simulink model "Horloge_interne_v3"  (R2023a)
settings: Solver=VariableStepAuto  StartTime=0.0  StopTime=20  RelTol=1e-3
settings Model: Creator=Khalid-B  LastModifiedBy=Khalid-B

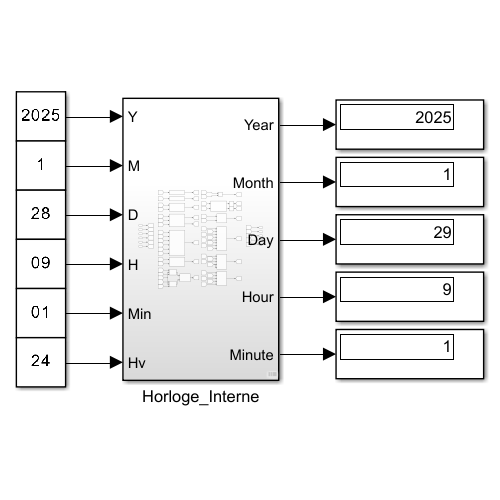
[thumbnail: Simulink's stored preview of the top-level diagram]
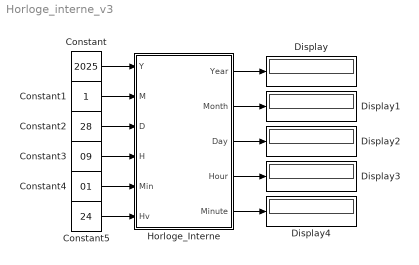
== system Horloge_interne_v3 ==
  Constant : Constant  Value=2025  OutDataTypeStr=uint32
  Constant1 : Constant  OutDataTypeStr=uint32
  Constant2 : Constant  Value=28  OutDataTypeStr=uint32
  Constant3 : Constant  Value=09  OutDataTypeStr=uint32
  Constant4 : Constant  Value=01  OutDataTypeStr=uint32
  Constant5 : Constant  Value=24  OutDataTypeStr=uint32
  Display{,1..4} (5 alike) : Display
  Horloge_Interne : Subsystem
  wires:
  Constant4/1 -> Horloge_Interne/5(Min)
  Constant2/1 -> Horloge_Interne/3(D)
  Horloge_Interne/4(Hour) -> Display3/1
  Horloge_Interne/2(Month) -> Display1/1
  Constant/1 -> Horloge_Interne/1(Y)
  Constant1/1 -> Horloge_Interne/2(M)
  Constant3/1 -> Horloge_Interne/4(H)
  Horloge_Interne/5(Minute) -> Display4/1
  Horloge_Interne/3(Day) -> Display2/1
  Horloge_Interne/1(Year) -> Display/1
  Constant5/1 -> Horloge_Interne/6(Hv)

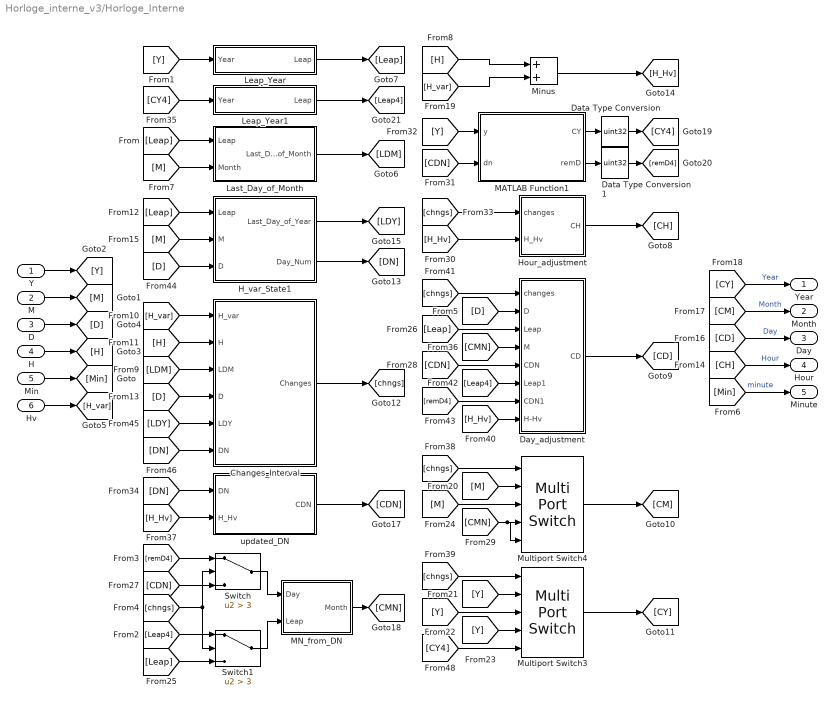
== system Horloge_interne_v3/Horloge_Interne ==
  Y : Inport
  M : Inport  Port=2
  D : Inport  Port=3
  H : Inport  Port=4
  Min : Inport  Port=5
  Hv : Inport  Port=6
  Changes_Interval : Subsystem
  Data Type Conversion : DataTypeConversion  OutDataTypeStr=uint32  SaturateOnIntegerOverflow=off  RndMeth=Floor
  Data Type Conversion1 : DataTypeConversion  OutDataTypeStr=uint32  SaturateOnIntegerOverflow=off  RndMeth=Floor
  Day_adjustment : Subsystem
  H_var_State1 : Subsystem
  Hour_adjustment : Subsystem
  Last_Day_of_Month : Subsystem
  Leap_Year : Subsystem
  Leap_Year1 : Subsystem
  MATLAB Function1 : MATLAB Function  TreatAsAtomicUnit=on
  MN_from_DN : Subsystem
  Minus : Sum
  Multiport Switch3 : MultiPortSwitch  Inputs=4  SaturateOnIntegerOverflow=off  InputSameDT=off
  Multiport Switch4 : MultiPortSwitch  Inputs=4  SaturateOnIntegerOverflow=off  InputSameDT=off
  Switch : Switch  Criteria=u2 > Threshold  Threshold=3  SaturateOnIntegerOverflow=off  InputSameDT=off
  Switch1 : Switch  Criteria=u2 > Threshold  Threshold=3  SaturateOnIntegerOverflow=off  InputSameDT=off
  updated_DN : Subsystem
  Year : Outport
  Month : Outport  Port=2
  Day : Outport  Port=3
  Hour : Outport  Port=4
  Minute : Outport  Port=5
  wires:
  updated_DN/1(CDN) -> [CDN]
  [CMN] -> Day_adjustment/4(M)
  [D] -> Day_adjustment/2(D)
  D/1 -> [D]
  [M] -> Last_Day_of_Month/2(Month)
  [H_Hv] -> Hour_adjustment/2(H_Hv)
  [H_Hv] -> updated_DN/2(H_Hv)
  [Y] -> Multiport Switch3/4
  [D] -> Changes_Interval/4(D)
  [Leap] -> H_var_State1/1(Leap)
  [CDN] -> Switch/3
  [H] -> Changes_Interval/2(H)
  M/1 -> [M]
  [Leap4] -> Switch1/1
  [chngs] -> Multiport Switch3/1
  [CDN] -> Day_adjustment/5(CDN)
  MATLAB Function1/1(CY) -> Data Type Conversion/1
  [Leap] -> Day_adjustment/3(Leap)
  [Y] -> Multiport Switch3/3
  MATLAB Function1/2(remD) -> Data Type Conversion1/1
  Changes_Interval/1(Changes) -> [chngs]
  Min/1 -> [Min]
  Multiport Switch4/1 -> [CM]
  [Leap4] -> Day_adjustment/6(Leap1)
  [H_var] -> Changes_Interval/1(H_var)
  Multiport Switch3/1 -> [CY]
  [remD4] -> Day_adjustment/7(CDN1)
  [CMN] -> Multiport Switch4/5, Multiport Switch4/4
  [chngs] -> Day_adjustment/1(changes)
  [chngs] -> Multiport Switch4/1
  [M] -> H_var_State1/2(M)
  [LDM] -> Changes_Interval/3(LDM)
  [Y] -> Multiport Switch3/2
  Last_Day_of_Month/1(Last_Day_of_Month) -> [LDM]
  [chngs] -> Switch/2, Switch1/2
  [M] -> Multiport Switch4/3
  [Leap] -> Switch1/3
  [DN] -> updated_DN/1(DN)
  [CDN] -> MATLAB Function1/2(dn)
  [M] -> Multiport Switch4/2
  MN_from_DN/1(Month) -> [CMN]
  [CY4] -> Multiport Switch3/5
  [Y] -> MATLAB Function1/1(y)
  Data Type Conversion1/1 -> [remD4]
  Day_adjustment/1(CD) -> [CD]
  [chngs] -> Hour_adjustment/1(changes)
  Hour_adjustment/1(CH) -> [CH]
  Data Type Conversion/1 -> [CY4]
  [remD4] -> Switch/1
  Y/1 -> [Y]
  [H_Hv] -> Day_adjustment/8(H-Hv)
  [Leap] -> Last_Day_of_Month/1(Leap)
  [CY] -> Year/1  "Year"
  [CM] -> Month/1  "Month"
  Hv/1 -> [H_var]
  [Min] -> Minute/1  "minute"
  H/1 -> [H]
  [CH] -> Hour/1  "Hour"
  [CD] -> Day/1  "Day"
  Leap_Year/1(Leap) -> [Leap]
  [Y] -> Leap_Year/1(Year)
  Leap_Year1/1(Leap) -> [Leap4]
  [CY4] -> Leap_Year1/1(Year)
  Switch/1 -> MN_from_DN/1(Day)
  Switch1/1 -> MN_from_DN/2(Leap)
  [D] -> H_var_State1/3(D)
  H_var_State1/2(Day_Num) -> [DN]
  H_var_State1/1(Last_Day_of_Year) -> [LDY]
  [LDY] -> Changes_Interval/5(LDY)
  [DN] -> Changes_Interval/6(DN)
  [H] -> Minus/1
  Minus/1 -> [H_Hv]
  [H_var] -> Minus/2

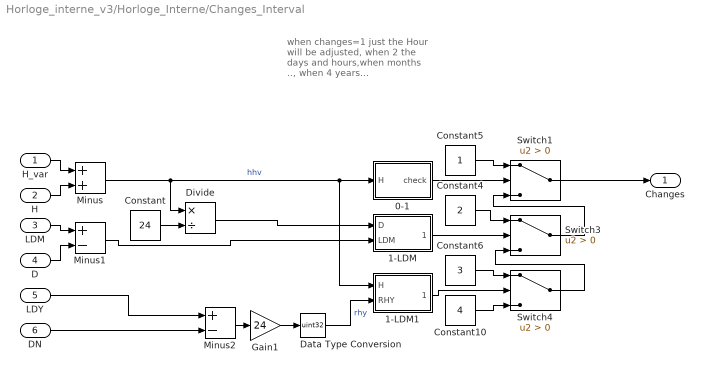
== system Horloge_interne_v3/Horloge_Interne/Changes_Interval ==
  note: when changes=1 just the Hour will be adjusted, when 2 the days and hours,when months .., when 4 years...
  H_var : Inport
  H : Inport  Port=2
  LDM : Inport  Port=3
  D : Inport  Port=4
  LDY : Inport  Port=5
  DN : Inport  Port=6
  0-1 : Subsystem
  1-LDM : Subsystem
  1-LDM1 : Subsystem
  Constant : Constant  Value=24  OutDataTypeStr=uint32
  Constant10 : Constant  Value=4  OutDataTypeStr=uint32
  Constant4 : Constant  Value=2  OutDataTypeStr=uint32
  Constant5 : Constant  OutDataTypeStr=uint32
  Constant6 : Constant  Value=3  OutDataTypeStr=uint32
  Data Type Conversion : DataTypeConversion  OutDataTypeStr=uint32  SaturateOnIntegerOverflow=off  RndMeth=Floor
  Divide : Product  Inputs=*/
  Gain1 : Gain  Gain=24
  Minus : Sum
  Minus1 : Sum  Inputs=+-
  Minus2 : Sum  Inputs=+-
  Switch1 : Switch  Criteria=u2 > Threshold  SaturateOnIntegerOverflow=off  InputSameDT=off
  Switch3 : Switch  Criteria=u2 > Threshold  SaturateOnIntegerOverflow=off  InputSameDT=off
  Switch4 : Switch  Criteria=u2 > Threshold  SaturateOnIntegerOverflow=off  InputSameDT=off
  Changes : Outport
  wires:
  Constant6/1 -> Switch4/1
  0-1/1(check) -> Switch1/2
  Constant5/1 -> Switch1/1
  Constant4/1 -> Switch3/1
  1-LDM/1(check) -> Switch3/2
  Minus/1 -> Divide/1, 0-1/1(H), 1-LDM1/1(H)  "hhv"
  Switch4/1 -> Switch3/3
  H/1 -> Minus/2
  1-LDM1/1(check) -> Switch4/2
  Constant10/1 -> Switch4/3
  Switch3/1 -> Switch1/3
  LDM/1 -> Minus1/1
  Minus2/1 -> Gain1/1
  H_var/1 -> Minus/1
  Switch1/1 -> Changes/1
  Constant/1 -> Divide/2
  Divide/1 -> 1-LDM/1(D)
  Data Type Conversion/1 -> 1-LDM1/2(RHY)  "rhy"
  Minus1/1 -> 1-LDM/2(LDM)
  Gain1/1 -> Data Type Conversion/1
  D/1 -> Minus1/2
  LDY/1 -> Minus2/1
  DN/1 -> Minus2/2

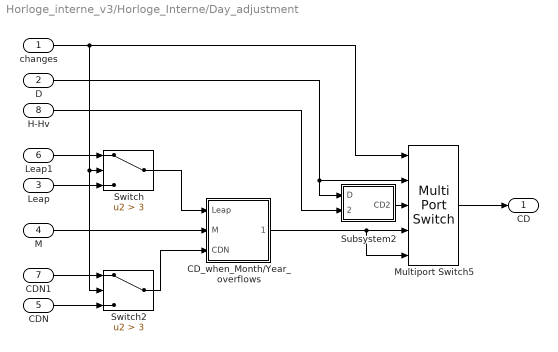
== system Horloge_interne_v3/Horloge_Interne/Day_adjustment ==
  changes : Inport
  D : Inport  Port=2
  Leap : Inport  Port=3
  M : Inport  Port=4
  CDN : Inport  Port=5
  Leap1 : Inport  Port=6
  CDN1 : Inport  Port=7
  H-Hv : Inport  Port=8
  CD_when_Month/Year_overflows : Subsystem
  Multiport Switch5 : MultiPortSwitch  Inputs=4  SaturateOnIntegerOverflow=off  InputSameDT=off
  Subsystem2 : Subsystem
  Switch : Switch  Criteria=u2 > Threshold  Threshold=3  SaturateOnIntegerOverflow=off  InputSameDT=off
  Switch2 : Switch  Criteria=u2 > Threshold  Threshold=3  SaturateOnIntegerOverflow=off  InputSameDT=off
  CD : Outport
  wires:
  changes/1 -> Switch2/2, Switch/2, Multiport Switch5/1
  Subsystem2/1(CD2) -> Multiport Switch5/3
  Multiport Switch5/1 -> CD/1
  D/1 -> Subsystem2/1(D), Multiport Switch5/2
  H-Hv/1 -> Subsystem2/2(H_Hv)
  CD_when_Month/Year_overflows/1(CD3_4) -> Multiport Switch5/5, Multiport Switch5/4
  Leap1/1 -> Switch/1
  Leap/1 -> Switch/3
  CDN1/1 -> Switch2/1
  CDN/1 -> Switch2/3
  M/1 -> CD_when_Month/Year_overflows/2(M)
  Switch/1 -> CD_when_Month/Year_overflows/1(Leap)
  Switch2/1 -> CD_when_Month/Year_overflows/3(CDN)

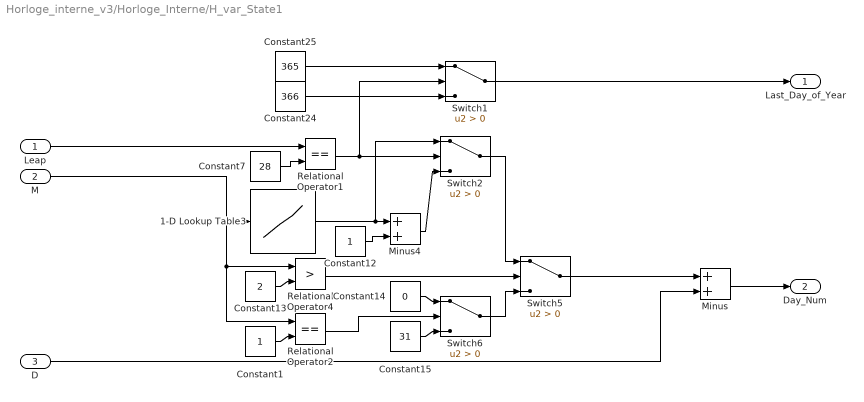
== system Horloge_interne_v3/Horloge_Interne/H_var_State1 ==
  Leap : Inport
  M : Inport  Port=2
  D : Inport  Port=3
  1-D Lookup Table3 : Lookup_n-D  NumberOfTableDimensions=1  BreakpointsSpecification=Even spacing  BreakpointsForDimension1=[-5:5]  Table=[0 0 59 90 120 151 181 212 243 273 304 334]  InterpMethod=Flat  InternalRulePriority=Speed  RndMeth=Simplest
  Constant1 : Constant  OutDataTypeStr=uint32
  Constant12 : Constant  OutDataTypeStr=uint32
  Constant13 : Constant  Value=2  OutDataTypeStr=uint32
  Constant14 : Constant  Value=0  OutDataTypeStr=uint32
  Constant15 : Constant  Value=31  OutDataTypeStr=uint32
  Constant24 : Constant  Value=366  OutDataTypeStr=uint32
  Constant25 : Constant  Value=365  OutDataTypeStr=uint32
  Constant7 : Constant  Value=28  OutDataTypeStr=uint32
  Minus : Sum
  Minus4 : Sum
  Relational Operator1 : RelationalOperator  Operator===  OutDataTypeStr=boolean  RndMeth=Simplest  InputSameDT=off
  Relational Operator2 : RelationalOperator  Operator===  OutDataTypeStr=boolean  RndMeth=Simplest  InputSameDT=off
  Relational Operator4 : RelationalOperator  Operator=>  OutDataTypeStr=boolean  RndMeth=Simplest  InputSameDT=off
  Switch{1..2,5..6} (4 alike) : Switch  Criteria=u2 > Threshold  SaturateOnIntegerOverflow=off  InputSameDT=off
  Last_Day_of_Year : Outport
  Day_Num : Outport  Port=2
  wires:
  M/1 -> Relational Operator2/1, Relational Operator4/1, 1-D Lookup Table3/1
  Switch1/1 -> Last_Day_of_Year/1
  Constant24/1 -> Switch1/3
  Constant25/1 -> Switch1/1
  Switch5/1 -> Minus/1
  D/1 -> Minus/2
  Minus/1 -> Day_Num/1
  Constant15/1 -> Switch6/3
  Constant12/1 -> Minus4/2
  Relational Operator4/1 -> Switch5/2
  Minus4/1 -> Switch2/3
  Switch2/1 -> Switch5/1
  Relational Operator1/1 -> Switch2/2, Switch1/2
  Constant13/1 -> Relational Operator4/2
  1-D Lookup Table3/1 -> Switch2/1, Minus4/1
  Constant7/1 -> Relational Operator1/2
  Switch6/1 -> Switch5/3
  Constant14/1 -> Switch6/1
  Leap/1 -> Relational Operator1/1
  Constant1/1 -> Relational Operator2/2
  Relational Operator2/1 -> Switch6/2

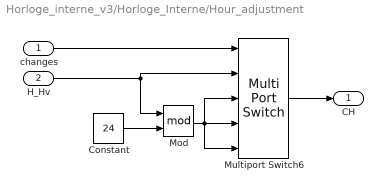
== system Horloge_interne_v3/Horloge_Interne/Hour_adjustment ==
  changes : Inport
  H_Hv : Inport  Port=2
  Constant : Constant  Value=24  OutDataTypeStr=uint32
  Mod : Math  Operator=mod
  Multiport Switch6 : MultiPortSwitch  Inputs=4  SaturateOnIntegerOverflow=off  InputSameDT=off
  CH : Outport
  wires:
  Multiport Switch6/1 -> CH/1
  H_Hv/1 -> Mod/1, Multiport Switch6/2
  Constant/1 -> Mod/2
  Mod/1 -> Multiport Switch6/5, Multiport Switch6/3, Multiport Switch6/4
  changes/1 -> Multiport Switch6/1

== system Horloge_interne_v3/Horloge_Interne/Last_Day_of_Month ==
  Leap : Inport
  Month : Inport  Port=2
  1-D Lookup Table : Lookup_n-D  NumberOfTableDimensions=1  LookupTableObject=obj1  BreakpointsSpecification=Even spacing  BreakpointsForDimension1=[1 3 5 6]  Table=[31 28 31 30 31 30 31 31 30 31 30 31]  InterpMethod=Flat  InternalRulePriority=Speed  RndMeth=Simplest
  Switch : Switch  Criteria=u2 > Threshold  Threshold=28  SaturateOnIntegerOverflow=off  InputSameDT=off
  Last_Day_of_Month : Outport
  wires:
  Leap/1 -> Switch/1, Switch/2
  Month/1 -> 1-D Lookup Table/1
  Switch/1 -> Last_Day_of_Month/1  "Last_Day_of_Month"
  1-D Lookup Table/1 -> Switch/3

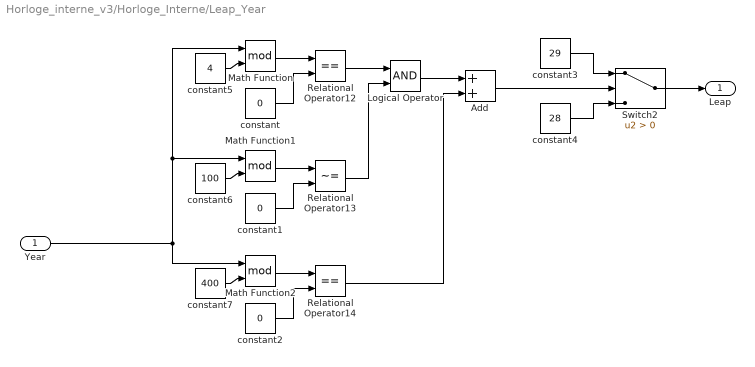
== system Horloge_interne_v3/Horloge_Interne/Leap_Year ==
  Year : Inport
  Add : Sum
  Logical Operator : Logic  AllPortsSameDT=off  OutDataTypeStr=boolean
  Math Function : Math  Operator=mod
  Math Function1 : Math  Operator=mod
  Math Function2 : Math  Operator=mod
  Relational Operator12 : RelationalOperator  Operator===  OutDataTypeStr=boolean  RndMeth=Simplest  InputSameDT=off
  Relational Operator13 : RelationalOperator  Operator=~=  OutDataTypeStr=boolean  RndMeth=Simplest  InputSameDT=off
  Relational Operator14 : RelationalOperator  Operator===  OutDataTypeStr=boolean  RndMeth=Simplest  InputSameDT=off
  Switch2 : Switch  Criteria=u2 > Threshold  SaturateOnIntegerOverflow=off  InputSameDT=off
  constant : Constant  Value=0  OutDataTypeStr=uint32
  constant1 : Constant  Value=0  OutDataTypeStr=uint32
  constant2 : Constant  Value=0  OutDataTypeStr=uint32
  constant3 : Constant  Value=29  OutDataTypeStr=uint32
  constant4 : Constant  Value=28  OutDataTypeStr=uint32
  constant5 : Constant  Value=4  OutDataTypeStr=uint32
  constant6 : Constant  Value=100  OutDataTypeStr=uint32
  constant7 : Constant  Value=400  OutDataTypeStr=uint32
  Leap : Outport
  wires:
  constant/1 -> Relational Operator12/2
  constant4/1 -> Switch2/3
  Year/1 -> Math Function2/1, Math Function1/1, Math Function/1
  Switch2/1 -> Leap/1
  Math Function2/1 -> Relational Operator14/1
  Relational Operator12/1 -> Logical Operator/1
  constant5/1 -> Math Function/2
  Relational Operator14/1 -> Add/2
  constant2/1 -> Relational Operator14/2
  Math Function/1 -> Relational Operator12/1
  Logical Operator/1 -> Add/1
  constant1/1 -> Relational Operator13/2
  Add/1 -> Switch2/2
  Relational Operator13/1 -> Logical Operator/2
  constant3/1 -> Switch2/1
  constant6/1 -> Math Function1/2
  constant7/1 -> Math Function2/2
  Math Function1/1 -> Relational Operator13/1

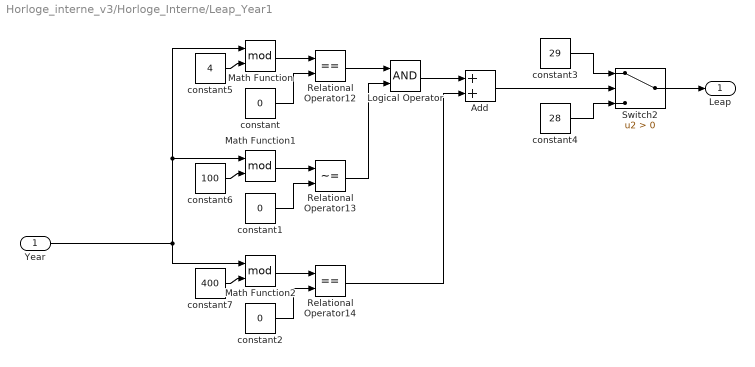
== system Horloge_interne_v3/Horloge_Interne/Leap_Year1 ==
  Year : Inport
  Add : Sum
  Logical Operator : Logic  AllPortsSameDT=off  OutDataTypeStr=boolean
  Math Function : Math  Operator=mod
  Math Function1 : Math  Operator=mod
  Math Function2 : Math  Operator=mod
  Relational Operator12 : RelationalOperator  Operator===  OutDataTypeStr=boolean  RndMeth=Simplest  InputSameDT=off
  Relational Operator13 : RelationalOperator  Operator=~=  OutDataTypeStr=boolean  RndMeth=Simplest  InputSameDT=off
  Relational Operator14 : RelationalOperator  Operator===  OutDataTypeStr=boolean  RndMeth=Simplest  InputSameDT=off
  Switch2 : Switch  Criteria=u2 > Threshold  SaturateOnIntegerOverflow=off  InputSameDT=off
  constant : Constant  Value=0  OutDataTypeStr=uint32
  constant1 : Constant  Value=0  OutDataTypeStr=uint32
  constant2 : Constant  Value=0  OutDataTypeStr=uint32
  constant3 : Constant  Value=29  OutDataTypeStr=uint32
  constant4 : Constant  Value=28  OutDataTypeStr=uint32
  constant5 : Constant  Value=4  OutDataTypeStr=uint32
  constant6 : Constant  Value=100  OutDataTypeStr=uint32
  constant7 : Constant  Value=400  OutDataTypeStr=uint32
  Leap : Outport
  wires:
  constant/1 -> Relational Operator12/2
  constant4/1 -> Switch2/3
  Year/1 -> Math Function2/1, Math Function1/1, Math Function/1
  Switch2/1 -> Leap/1
  Math Function2/1 -> Relational Operator14/1
  Relational Operator12/1 -> Logical Operator/1
  constant5/1 -> Math Function/2
  Relational Operator14/1 -> Add/2
  constant2/1 -> Relational Operator14/2
  Math Function/1 -> Relational Operator12/1
  Logical Operator/1 -> Add/1
  constant1/1 -> Relational Operator13/2
  Add/1 -> Switch2/2
  Relational Operator13/1 -> Logical Operator/2
  constant3/1 -> Switch2/1
  constant6/1 -> Math Function1/2
  constant7/1 -> Math Function2/2
  Math Function1/1 -> Relational Operator13/1

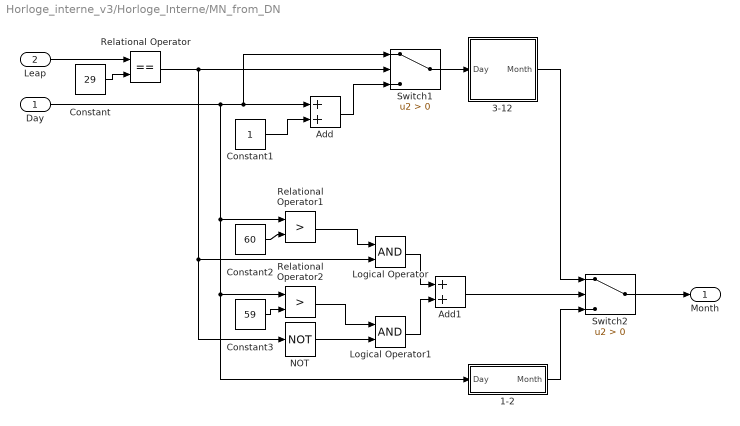
== system Horloge_interne_v3/Horloge_Interne/MN_from_DN ==
  Day : Inport
  Leap : Inport  Port=2
  1-2 : Subsystem
  3-12 : Subsystem
  Add : Sum
  Add1 : Sum
  Constant : Constant  Value=29  OutDataTypeStr=uint32
  Constant1 : Constant  OutDataTypeStr=uint32
  Constant2 : Constant  Value=60  OutDataTypeStr=uint32
  Constant3 : Constant  Value=59  OutDataTypeStr=uint32
  Logical Operator : Logic  AllPortsSameDT=off  OutDataTypeStr=boolean
  Logical Operator1 : Logic  AllPortsSameDT=off  OutDataTypeStr=boolean
  NOT : Logic  Operator=NOT  IconShape=distinctive  AllPortsSameDT=off  OutDataTypeStr=boolean
  Relational Operator : RelationalOperator  Operator===  OutDataTypeStr=boolean  RndMeth=Simplest  InputSameDT=off
  Relational Operator1 : RelationalOperator  Operator=>  OutDataTypeStr=boolean  RndMeth=Simplest  InputSameDT=off
  Relational Operator2 : RelationalOperator  Operator=>  OutDataTypeStr=boolean  RndMeth=Simplest  InputSameDT=off
  Switch1 : Switch  Criteria=u2 > Threshold  SaturateOnIntegerOverflow=off  InputSameDT=off
  Switch2 : Switch  Criteria=u2 > Threshold  SaturateOnIntegerOverflow=off  InputSameDT=off
  Month : Outport
  wires:
  Constant/1 -> Relational Operator/2
  Switch1/1 -> 3-12/1(Day)
  Add/1 -> Switch1/3
  Constant1/1 -> Add/2
  Constant2/1 -> Relational Operator1/2
  Relational Operator1/1 -> Logical Operator/1
  Constant3/1 -> Relational Operator2/2
  Relational Operator2/1 -> Logical Operator1/1
  Day/1 -> 1-2/1(Day), Relational Operator2/1, Relational Operator1/1, Switch1/1, Add/1
  Relational Operator/1 -> NOT/1, Logical Operator/2, Switch1/2
  Logical Operator/1 -> Add1/1
  Logical Operator1/1 -> Add1/2
  Add1/1 -> Switch2/2
  3-12/1(Month) -> Switch2/1
  1-2/1(Month) -> Switch2/3
  Switch2/1 -> Month/1
  Leap/1 -> Relational Operator/1
  NOT/1 -> Logical Operator1/2

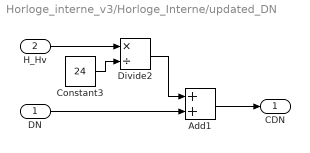
== system Horloge_interne_v3/Horloge_Interne/updated_DN ==
  DN : Inport
  H_Hv : Inport  Port=2
  Add1 : Sum
  Constant3 : Constant  Value=24  OutDataTypeStr=uint32
  Divide2 : Product  Inputs=*/
  CDN : Outport
  wires:
  Constant3/1 -> Divide2/2
  Divide2/1 -> Add1/1
  H_Hv/1 -> Divide2/1
  DN/1 -> Add1/2
  Add1/1 -> CDN/1

== system Horloge_interne_v3/Horloge_Interne/Changes_Interval/0-1 ==
  H : Inport
  Constant1 : Constant  Value=24  OutDataTypeStr=uint32
  Relational Operator1 : RelationalOperator  Operator=<  OutDataTypeStr=boolean  RndMeth=Simplest  InputSameDT=off
  check : Outport
  wires:
  Relational Operator1/1 -> check/1
  H/1 -> Relational Operator1/1
  Constant1/1 -> Relational Operator1/2

== system Horloge_interne_v3/Horloge_Interne/Changes_Interval/1-LDM ==
  D : Inport
  LDM : Inport  Port=2
  Relational Operator : RelationalOperator  Operator=<=  OutDataTypeStr=boolean  RndMeth=Simplest  InputSameDT=off
  check : Outport
  wires:
  D/1 -> Relational Operator/1
  LDM/1 -> Relational Operator/2
  Relational Operator/1 -> check/1

== system Horloge_interne_v3/Horloge_Interne/Changes_Interval/1-LDM1 ==
  H : Inport
  RHY : Inport  Port=2
  Relational Operator : RelationalOperator  Operator=<  OutDataTypeStr=boolean  RndMeth=Simplest  InputSameDT=off
  check : Outport
  wires:
  Relational Operator/1 -> check/1
  H/1 -> Relational Operator/1
  RHY/1 -> Relational Operator/2

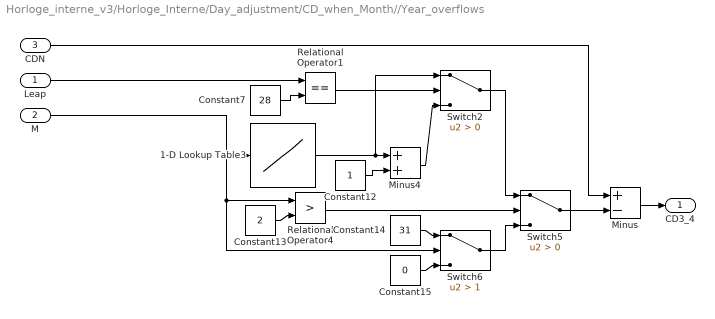
== system Horloge_interne_v3/Horloge_Interne/Day_adjustment/CD_when_Month//Year_overflows ==
  Leap : Inport
  M : Inport  Port=2
  CDN : Inport  Port=3
  1-D Lookup Table3 : Lookup_n-D  NumberOfTableDimensions=1  BreakpointsSpecification=Even spacing  BreakpointsForDimension1=[-5:5]  Table=[0 0 59 90 120 151 181 212 243 273 304 334]  InterpMethod=Flat  InternalRulePriority=Speed  RndMeth=Simplest
  Constant12 : Constant  OutDataTypeStr=uint32
  Constant13 : Constant  Value=2  OutDataTypeStr=uint32
  Constant14 : Constant  Value=31  OutDataTypeStr=uint32
  Constant15 : Constant  Value=0  OutDataTypeStr=uint32
  Constant7 : Constant  Value=28  OutDataTypeStr=uint32
  Minus : Sum  Inputs=+-
  Minus4 : Sum
  Relational Operator1 : RelationalOperator  Operator===  OutDataTypeStr=boolean  RndMeth=Simplest  InputSameDT=off
  Relational Operator4 : RelationalOperator  Operator=>  OutDataTypeStr=boolean  RndMeth=Simplest  InputSameDT=off
  Switch2 : Switch  Criteria=u2 > Threshold  SaturateOnIntegerOverflow=off  InputSameDT=off
  Switch5 : Switch  Criteria=u2 > Threshold  SaturateOnIntegerOverflow=off  InputSameDT=off
  Switch6 : Switch  Criteria=u2 > Threshold  Threshold=1  SaturateOnIntegerOverflow=off  InputSameDT=off
  CD3_4 : Outport
  wires:
  CDN/1 -> Minus/1
  Switch5/1 -> Minus/2
  Minus/1 -> CD3_4/1
  M/1 -> Switch6/2, Relational Operator4/1, 1-D Lookup Table3/1
  Leap/1 -> Relational Operator1/1
  Switch6/1 -> Switch5/3
  Constant14/1 -> Switch6/1
  1-D Lookup Table3/1 -> Switch2/1, Minus4/1
  Relational Operator4/1 -> Switch5/2
  Constant15/1 -> Switch6/3
  Constant12/1 -> Minus4/2
  Constant13/1 -> Relational Operator4/2
  Switch2/1 -> Switch5/1
  Minus4/1 -> Switch2/3
  Relational Operator1/1 -> Switch2/2
  Constant7/1 -> Relational Operator1/2

== system Horloge_interne_v3/Horloge_Interne/Day_adjustment/Subsystem2 ==
  D : Inport
  H_Hv : Inport  Port=2
  Add1 : Sum
  Constant3 : Constant  Value=24  OutDataTypeStr=uint32
  Divide1 : Product  Inputs=*/
  CD2 : Outport
  wires:
  H_Hv/1 -> Divide1/1
  Constant3/1 -> Divide1/2
  Add1/1 -> CD2/1
  D/1 -> Add1/1
  Divide1/1 -> Add1/2

== system Horloge_interne_v3/Horloge_Interne/MN_from_DN/1-2 ==
  Day : Inport
  1-31 : Subsystem
  Constant1 : Constant  Value=2  OutDataTypeStr=uint32
  Constant2 : Constant  OutDataTypeStr=uint32
  Switch2 : Switch  Criteria=u2 > Threshold  SaturateOnIntegerOverflow=off  InputSameDT=off
  Month : Outport
  wires:
  Constant2/1 -> Switch2/1
  Constant1/1 -> Switch2/3
  1-31/1(check) -> Switch2/2
  Day/1 -> 1-31/1(D)
  Switch2/1 -> Month/1

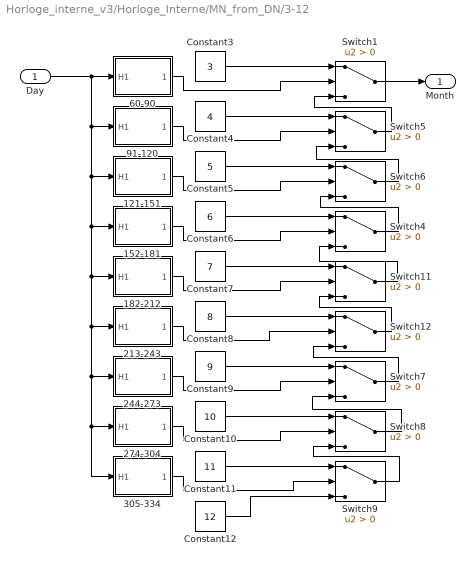
== system Horloge_interne_v3/Horloge_Interne/MN_from_DN/3-12 ==
  Day : Inport
  121-151 : Subsystem
  152-181 : Subsystem
  182-212 : Subsystem
  213-243 : Subsystem
  244-273 : Subsystem
  274-304 : Subsystem
  305-334 : Subsystem
  60-90 : Subsystem
  91-120 : Subsystem
  Constant10 : Constant  Value=10  OutDataTypeStr=uint32
  Constant11 : Constant  Value=11  OutDataTypeStr=uint32
  Constant12 : Constant  Value=12  OutDataTypeStr=uint32
  Constant3 : Constant  Value=3  OutDataTypeStr=uint32
  Constant4 : Constant  Value=4  OutDataTypeStr=uint32
  Constant5 : Constant  Value=5  OutDataTypeStr=uint32
  Constant6 : Constant  Value=6  OutDataTypeStr=uint32
  Constant7 : Constant  Value=7  OutDataTypeStr=uint32
  Constant8 : Constant  Value=8  OutDataTypeStr=uint32
  Constant9 : Constant  Value=9  OutDataTypeStr=uint32
  Switch{1,4..9,11..12} (9 alike) : Switch  Criteria=u2 > Threshold  SaturateOnIntegerOverflow=off  InputSameDT=off
  Month : Outport
  wires:
  Switch11/1 -> Switch4/3
  Constant10/1 -> Switch8/1
  Constant12/1 -> Switch9/3
  Switch5/1 -> Switch1/3
  Switch7/1 -> Switch12/3
  121-151/1(check1) -> Switch6/2
  182-212/1(check1) -> Switch11/2
  Switch8/1 -> Switch7/3
  Switch9/1 -> Switch8/3
  Constant4/1 -> Switch5/1
  Constant8/1 -> Switch12/1
  152-181/1(check1) -> Switch4/2
  Constant3/1 -> Switch1/1
  244-273/1(check1) -> Switch7/2
  Constant6/1 -> Switch4/1
  Constant9/1 -> Switch7/1
  Constant7/1 -> Switch11/1
  213-243/1(check1) -> Switch12/2
  Switch12/1 -> Switch11/3
  274-304/1(check1) -> Switch8/2
  Constant11/1 -> Switch9/1
  60-90/1(check1) -> Switch1/2
  Switch6/1 -> Switch5/3
  Switch4/1 -> Switch6/3
  305-334/1(check1) -> Switch9/2
  91-120/1(check1) -> Switch5/2
  Constant5/1 -> Switch6/1
  Day/1 -> 274-304/1(H1), 305-334/1(H1), 244-273/1(H1), 213-243/1(H1), 182-212/1(H1), 152-181/1(H1), 121-151/1(H1), 91-120/1(H1), 60-90/1(H1)
  Switch1/1 -> Month/1

== system Horloge_interne_v3/Horloge_Interne/MN_from_DN/1-2/1-31 ==
  D : Inport
  Constant1 : Constant  Value=31  OutDataTypeStr=uint32
  Relational Operator1 : RelationalOperator  Operator=<=  OutDataTypeStr=boolean  RndMeth=Simplest  InputSameDT=off
  check : Outport
  wires:
  Constant1/1 -> Relational Operator1/2
  Relational Operator1/1 -> check/1
  D/1 -> Relational Operator1/1

== system Horloge_interne_v3/Horloge_Interne/MN_from_DN/3-12/121-151 ==
  H1 : Inport
  Constant1 : Constant  Value=152  OutDataTypeStr=uint32
  Relational Operator1 : RelationalOperator  Operator=<=  OutDataTypeStr=boolean  RndMeth=Simplest  InputSameDT=off
  check1 : Outport
  wires:
  Relational Operator1/1 -> check1/1
  H1/1 -> Relational Operator1/1
  Constant1/1 -> Relational Operator1/2

== system Horloge_interne_v3/Horloge_Interne/MN_from_DN/3-12/152-181 ==
  H1 : Inport
  Constant1 : Constant  Value=182  OutDataTypeStr=uint32
  Relational Operator1 : RelationalOperator  Operator=<=  OutDataTypeStr=boolean  RndMeth=Simplest  InputSameDT=off
  check1 : Outport
  wires:
  Relational Operator1/1 -> check1/1
  H1/1 -> Relational Operator1/1
  Constant1/1 -> Relational Operator1/2

== system Horloge_interne_v3/Horloge_Interne/MN_from_DN/3-12/182-212 ==
  H1 : Inport
  Constant1 : Constant  Value=213  OutDataTypeStr=uint32
  Relational Operator1 : RelationalOperator  Operator=<=  OutDataTypeStr=boolean  RndMeth=Simplest  InputSameDT=off
  check1 : Outport
  wires:
  Relational Operator1/1 -> check1/1
  H1/1 -> Relational Operator1/1
  Constant1/1 -> Relational Operator1/2

== system Horloge_interne_v3/Horloge_Interne/MN_from_DN/3-12/213-243 ==
  H1 : Inport
  Constant1 : Constant  Value=244  OutDataTypeStr=uint32
  Relational Operator1 : RelationalOperator  Operator=<=  OutDataTypeStr=boolean  RndMeth=Simplest  InputSameDT=off
  check1 : Outport
  wires:
  Relational Operator1/1 -> check1/1
  H1/1 -> Relational Operator1/1
  Constant1/1 -> Relational Operator1/2

== system Horloge_interne_v3/Horloge_Interne/MN_from_DN/3-12/244-273 ==
  H1 : Inport
  Constant1 : Constant  Value=274  OutDataTypeStr=uint32
  Relational Operator1 : RelationalOperator  Operator=<=  OutDataTypeStr=boolean  RndMeth=Simplest  InputSameDT=off
  check1 : Outport
  wires:
  Relational Operator1/1 -> check1/1
  H1/1 -> Relational Operator1/1
  Constant1/1 -> Relational Operator1/2

== system Horloge_interne_v3/Horloge_Interne/MN_from_DN/3-12/274-304 ==
  H1 : Inport
  Constant1 : Constant  Value=305  OutDataTypeStr=uint32
  Relational Operator1 : RelationalOperator  Operator=<=  OutDataTypeStr=boolean  RndMeth=Simplest  InputSameDT=off
  check1 : Outport
  wires:
  Relational Operator1/1 -> check1/1
  H1/1 -> Relational Operator1/1
  Constant1/1 -> Relational Operator1/2

== system Horloge_interne_v3/Horloge_Interne/MN_from_DN/3-12/305-334 ==
  H1 : Inport
  Constant1 : Constant  Value=335  OutDataTypeStr=uint32
  Relational Operator1 : RelationalOperator  Operator=<=  OutDataTypeStr=boolean  RndMeth=Simplest  InputSameDT=off
  check1 : Outport
  wires:
  Relational Operator1/1 -> check1/1
  H1/1 -> Relational Operator1/1
  Constant1/1 -> Relational Operator1/2

== system Horloge_interne_v3/Horloge_Interne/MN_from_DN/3-12/60-90 ==
  H1 : Inport
  Constant1 : Constant  Value=91  OutDataTypeStr=uint32
  Relational Operator1 : RelationalOperator  Operator=<=  OutDataTypeStr=boolean  RndMeth=Simplest  InputSameDT=off
  check1 : Outport
  wires:
  H1/1 -> Relational Operator1/1
  Constant1/1 -> Relational Operator1/2
  Relational Operator1/1 -> check1/1

== system Horloge_interne_v3/Horloge_Interne/MN_from_DN/3-12/91-120 ==
  H1 : Inport
  Constant1 : Constant  Value=121  OutDataTypeStr=uint32
  Relational Operator1 : RelationalOperator  Operator=<=  OutDataTypeStr=boolean  RndMeth=Simplest  InputSameDT=off
  check1 : Outport
  wires:
  H1/1 -> Relational Operator1/1
  Constant1/1 -> Relational Operator1/2
  Relational Operator1/1 -> check1/1

== matlab function Horloge_interne_v3/Horloge_Interne/MATLAB Function1 ==
  data: y input; CY output; remD output; dn input
function [CY,remD] = case_4_function(y,dn)
y=int32(y);
dn=int32(dn);
remD=int32(dn);
CY=int32(0);
if dn >LDY(y)
while remD>LDY(y+CY)
    remD=remD-LDY(y+CY);
    CY=CY+int32(1);
end
end
CY=CY+y;
end


function [LD]=LDY(Year)
if mod(Year,4)==0 && mod(Year,100)~=0 || mod(Year,400)==0
    LD=int32(366);
else 
    LD=int32(365);
end
end
